simulink library "gensetMV"  (R2013a)
settings: Solver=ode3  StartTime=0.0  StopTime=10.0  RelTol=1e-3
values from neighbouring files (symbols this model uses):
  AFlowcontrol = AFhighc    (= 23)    [init_ele.m]
  AFn = 27*ones(engines,1)    [initHybrid.m]    (also in initMV.m; init_ele.m = 27)
  genset = generators(1)    [runTempCyl4S.m]
  i = i + 1    (= 2)    [DataProcessGUI1.m]    (also in NOxProcessGUI.m)
  ma0 = .2*ones(engines,1)    [initHybrid.m]    (also in initMV.m; init_ele.m = 0.2)
  nr = 1    [init_ele.m]
undefined symbols (not defined in the file or in its folder): generators, Kappa1, magnitude, pin0, swbId
libraries: goto x6, genset x2, EngineSysteSubmodel x2, simulink x1, switchboard x1
settings Model: Creator=torstebo  LastModifiedBy=yum

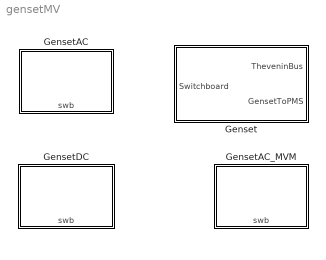
== system gensetMV ==
  Genset : Subsystem
  GensetAC : Subsystem  Tag=GensetAC  mask{genset=generators(6), swbId=3}
      mask prompts: genset "Generator set data"; swbId "SwitchboardId"
      mask Display: image(imread('figs/generator.jpg'),'center')
  GensetAC_MVM : Subsystem  Tag=GensetAC  mask{genset=generators(1), swbId=3}
      mask prompts: genset "Generator set data"; swbId "SwitchboardId"
      mask Display: image(imread('figs/generator.jpg'),'center')
  GensetDC : Subsystem  Tag=GensetDC  mask{genset=generators(1), swbId=1}
      mask prompts: genset "Generator set data"; swbId "SwitchboardId"
      mask Display: image(imread('figs/generator.jpg'),'center')

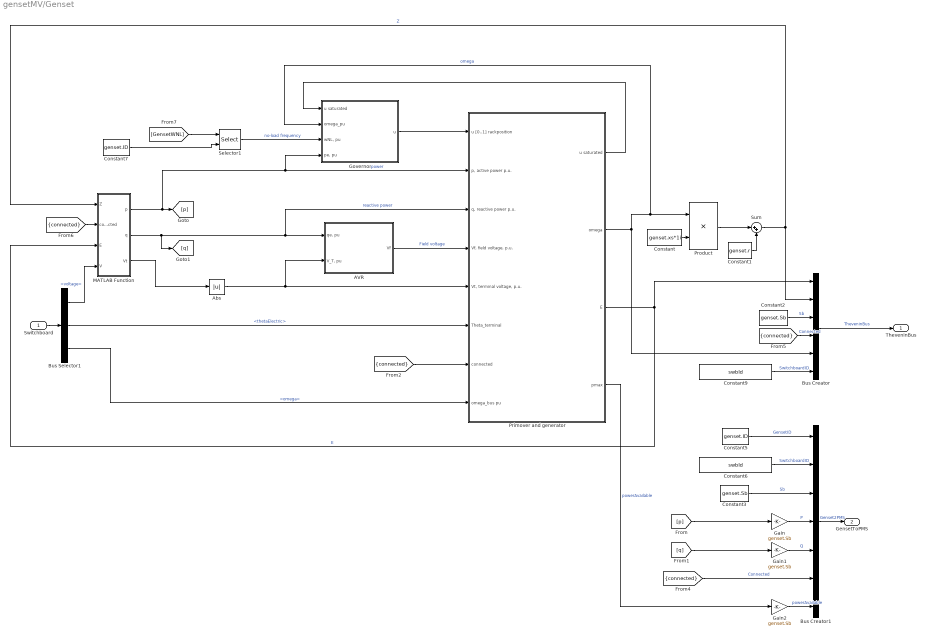
== system gensetMV/Genset ==
  Switchboard : Inport
  AVR : Subsystem
  Abs : Abs
  Bus Creator : BusCreator  Inputs='E','Z','Sb','Connected','omega','SwitchboardID'  OutDataTypeStr=Bus: TheveninBus  NonVirtualBus=on
  Bus Creator1 : BusCreator  Inputs='GensetID','SwitchboardID','Sb','P','Q','Connected','powerAvailable'  OutDataTypeStr=Bus: Genset2PMS  NonVirtualBus=on
  Bus Selector1 : BusSelector  OutputSignals=voltage,thetaElectric,omega
  Constant : Constant  Value=genset.xs*1i
  Constant1 : Constant  Value=genset.r
  Constant2 : Constant  Value=genset.Sb
  Constant3 : Constant  Value=genset.Sb
  Constant5 : Constant  Value=genset.ID  OutDataTypeStr=Inherit: Inherit via back propagation
  Constant6 : Constant  Value=swbId  OutDataTypeStr=Inherit: Inherit via back propagation
  Constant7 : Constant  Value=genset.ID  OutDataTypeStr=Inherit: Inherit via back propagation
  Constant9 : Constant  Value=swbId  OutDataTypeStr=Inherit: Inherit via back propagation
  Gain : Gain  Gain=genset.Sb
  Gain1 : Gain  Gain=genset.Sb
  Gain2 : Gain  Gain=genset.Sb
  Governor : Subsystem
  MATLAB Function : MATLAB Function  TreatAsAtomicUnit=on
  Primover and generator : Subsystem
  Product : Product
  Selector1 : Selector  IndexOptions=Index vector (port)  Indices=[nr]  OutputSizes=1
  Sum : Sum  Inputs=|++
  TheveninBus : Outport
  GensetToPMS : Outport  Port=2
  wires:
  Bus Selector1/2 -> Primover and generator/6(Theta_terminal)  "<thetaElectric>"
  Constant9/1 -> Bus Creator/6  "SwitchboardID"
  Switchboard/1 -> Bus Selector1/1
  Bus Selector1/3 -> Primover and generator/8(omega_bus pu)  "<omega>"
  MATLAB Function/3(Vt) -> Abs/1
  [connected] -> Bus Creator/4  "Connected"
  [connected] -> Bus Creator1/6  "Connected"
  [connected] -> MATLAB Function/2(connected)
  [connected] -> Primover and generator/7(connected)
  Gain2/1 -> Bus Creator1/7  "powerAvailable"
  Bus Selector1/1 -> MATLAB Function/4(V)  "<voltage>"
  Gain1/1 -> Bus Creator1/5  "Q"
  Gain/1 -> Bus Creator1/4  "P"
  Constant6/1 -> Bus Creator1/2  "SwitchboardID"
  Constant5/1 -> Bus Creator1/1  "GensetID"
  Constant3/1 -> Bus Creator1/3  "Sb"
  Selector1/1 -> Governor/3("wNL, pu")  "no-load frequency"
  AVR/1(Vf) -> Primover and generator/4("Vf, field voltage, p.u.")  "Field voltage"
  Primover and generator/1(u saturated) -> Governor/1(u saturated)
  Primover and generator/2(omega) -> Bus Creator/5, Governor/2(omega_pu), Product/1  "omega"
  Primover and generator/3(E) -> MATLAB Function/3(E), Bus Creator/1  "E"
  Governor/1(u) -> Primover and generator/1(u [0..1] rackposition)
  [GensetWNL] -> Selector1/1
  MATLAB Function/1(p) -> Primover and generator/2("p, active power p.u."), Governor/4("pe, pu"), [p]  "power"
  MATLAB Function/2(q) -> Primover and generator/3("q, reactive power p.u."), AVR/1("qe, pu"), [q]  "reactive power"
  Primover and generator/4(pmax) -> Gain2/1  "powerAvailable"
  Abs/1 -> Primover and generator/5("Vt, terminal voltage, p.u."), AVR/2("V_T, pu")
  Constant/1 -> Product/2
  Product/1 -> Sum/1
  Constant1/1 -> Sum/2
  Sum/1 -> MATLAB Function/1(Z), Bus Creator/2  "Z"
  Bus Creator/1 -> TheveninBus/1  "TheveninBus"
  Constant2/1 -> Bus Creator/3  "Sb"
  [q] -> Gain1/1
  [p] -> Gain/1
  Constant7/1 -> Selector1/2
  Bus Creator1/1 -> GensetToPMS/1  "Genset2PMS"

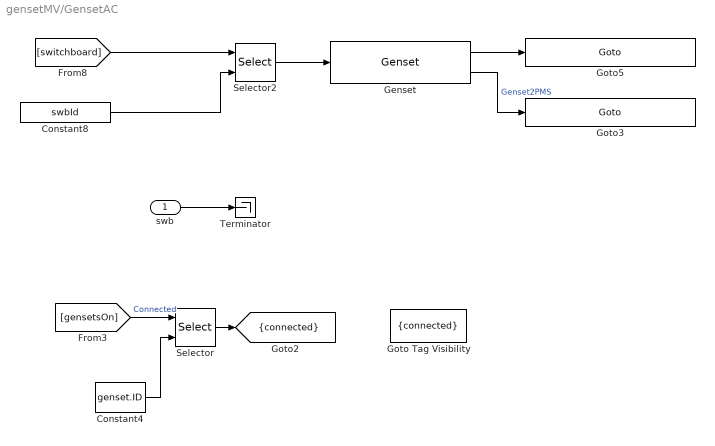
== system gensetMV/GensetAC ==
  swb : Inport
  Constant4 : Constant  Value=genset.ID  OutDataTypeStr=Inherit: Inherit via back propagation
  Constant8 : Constant  Value=swbId  OutDataTypeStr=Inherit: Inherit via back propagation
  Genset : genset/Genset
  Goto Tag Visibility : GotoTagVisibility  GotoTag=connected
  Goto3 : goto/Goto  GotoTag=sprintf('Generatorset%d',genset.ID)
  Goto5 : goto/Goto  GotoTag=sprintf('GeneratorsetElectric%d',genset.ID)
  Selector : Selector  IndexOptions=Index vector (port)  Indices=[nr]  OutputSizes=1
  Selector2 : Selector  IndexOptions=Index vector (port)  Indices=[nr]  OutputSizes=1
  Terminator : Terminator
  tag scope: connected=scoped
  wires:
  Constant8/1 -> Selector2/2
  swb/1 -> Terminator/1
  Selector/1 -> [connected]
  [gensetsOn] -> Selector/1  "Connected"
  [switchboard] -> Selector2/1
  Constant4/1 -> Selector/2
  Selector2/1 -> Genset/1
  Genset/1 -> Goto5/1
  Genset/2 -> Goto3/1  "Genset2PMS"

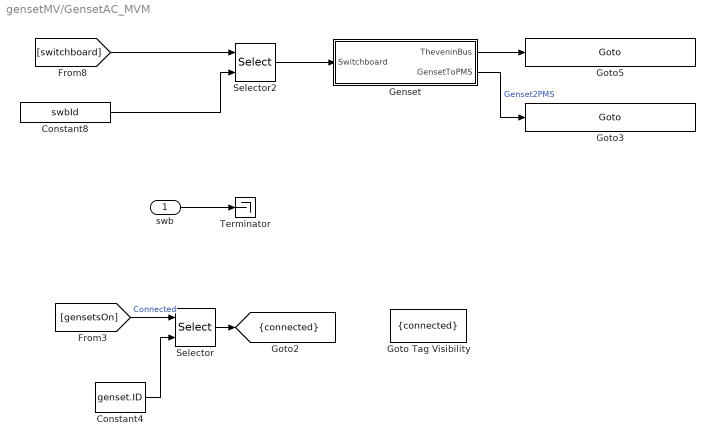
== system gensetMV/GensetAC_MVM ==
  swb : Inport
  Constant4 : Constant  Value=genset.ID  OutDataTypeStr=Inherit: Inherit via back propagation
  Constant8 : Constant  Value=swbId  OutDataTypeStr=Inherit: Inherit via back propagation
  Genset : Subsystem
  Goto Tag Visibility : GotoTagVisibility  GotoTag=connected
  Goto3 : goto/Goto  GotoTag=sprintf('Generatorset%d',genset.ID)
  Goto5 : goto/Goto  GotoTag=sprintf('GeneratorsetElectric%d',genset.ID)
  Selector : Selector  IndexOptions=Index vector (port)  Indices=[nr]  OutputSizes=1
  Selector2 : Selector  IndexOptions=Index vector (port)  Indices=[nr]  OutputSizes=1
  Terminator : Terminator
  tag scope: connected=scoped
  wires:
  Constant8/1 -> Selector2/2
  swb/1 -> Terminator/1
  Selector/1 -> [connected]
  [gensetsOn] -> Selector/1  "Connected"
  [switchboard] -> Selector2/1
  Constant4/1 -> Selector/2
  Selector2/1 -> Genset/1(Switchboard)
  Genset/1(TheveninBus) -> Goto5/1
  Genset/2(GensetToPMS) -> Goto3/1  "Genset2PMS"

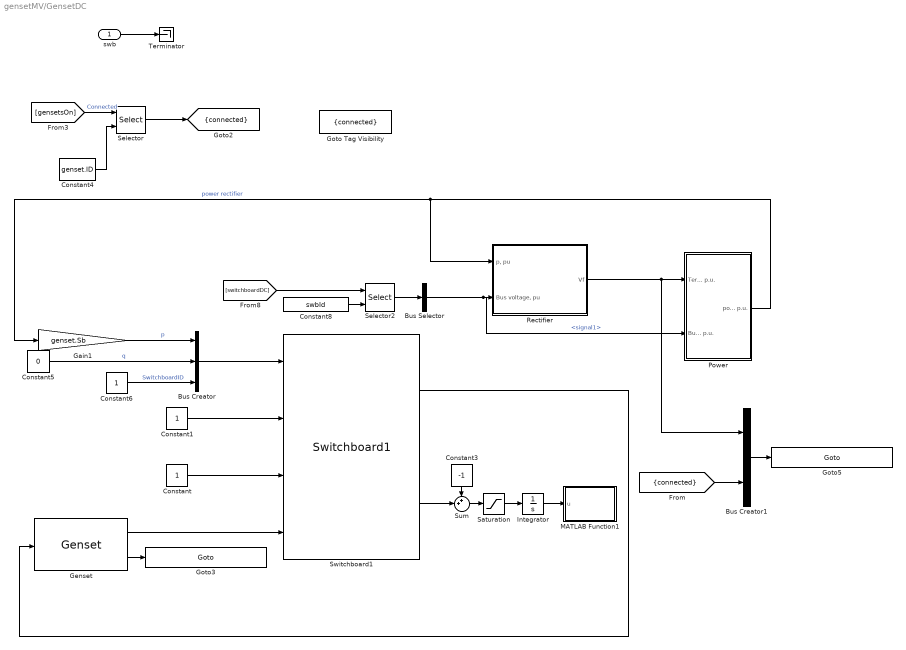
== system gensetMV/GensetDC ==
  swb : Inport
  Bus Creator : BusCreator  Inputs=3  OutDataTypeStr=Bus: powerLoadsBus
  Bus Creator1 : BusCreator  Inputs=2
  Bus Selector : BusSelector  OutputSignals=signal1
  Constant : Constant
  Constant1 : Constant
  Constant3 : Constant  Value=-1
  Constant4 : Constant  Value=genset.ID  OutDataTypeStr=Inherit: Inherit via back propagation
  Constant5 : Constant  Value=0
  Constant6 : Constant
  Constant8 : Constant  Value=swbId  OutDataTypeStr=Inherit: Inherit via back propagation
  Gain1 : Gain  Gain=genset.Sb
  Genset : genset/Genset
  Goto Tag Visibility : GotoTagVisibility  GotoTag=connected
  Goto3 : goto/Goto  GotoTag=sprintf('GeneratorsetDC%d',genset.ID)
  Goto5 : goto/Goto  GotoTag=sprintf('GeneratorsetElectricDC%d',genset.ID)
  Integrator : Integrator
  MATLAB Function1 : MATLAB Function  TreatAsAtomicUnit=on
  Power : Subsystem
  Rectifier : Subsystem
  Saturation : Saturate  UpperLimit=0  LowerLimit=-1
  Selector : Selector  IndexOptions=Index vector (port)  Indices=[nr]  OutputSizes=1
  Selector2 : Selector  IndexOptions=Index vector (port)  Indices=[nr]  OutputSizes=1
  Sum : Sum  Inputs=++|
  Switchboard1 : switchboard/Switchboard1
  Terminator : Terminator
  tag scope: connected=scoped
  wires:
  Constant8/1 -> Selector2/2
  swb/1 -> Terminator/1
  Selector/1 -> [connected]
  [gensetsOn] -> Selector/1  "Connected"
  [switchboardDC] -> Selector2/1
  Constant4/1 -> Selector/2
  Selector2/1 -> Bus Selector/1
  Rectifier/1(Vf) -> Bus Creator1/1, Power/1(Terminal Voltage p.u.)
  Power/1(power p.u.) -> Rectifier/1("p, pu"), Gain1/1  "power rectifier"
  Bus Selector/1 -> Power/2(Bus Voltage p.u.), Rectifier/2("Bus voltage, pu")  "<signal1>"
  Gain1/1 -> Bus Creator/1  "p"
  Bus Creator/1 -> Switchboard1/1
  Constant3/1 -> Sum/1
  Constant5/1 -> Bus Creator/2  "q"
  Integrator/1 -> MATLAB Function1/1(u)
  Genset/1 -> Switchboard1/4
  Constant/1 -> Switchboard1/3
  Sum/1 -> Saturation/1
  Saturation/1 -> Integrator/1
  Switchboard1/1 -> Genset/1
  Constant6/1 -> Bus Creator/3  "SwitchboardID"
  Switchboard1/2 -> Sum/2
  Constant1/1 -> Switchboard1/2
  Bus Creator1/1 -> Goto5/1
  [connected] -> Bus Creator1/2
  Genset/2 -> Goto3/1

== system gensetMV/Genset/AVR ==
  "qe, pu" : Inport
  "V_T, pu" : Inport  Port=2
  Constant : Constant
  Constant7 : Constant  Value=genset.ID  OutDataTypeStr=Inherit: Inherit via back propagation
  Gain : Gain  Gain=genset.avr.droop
  Low pass filter : Subsystem
  PI controller : Subsystem
  Product : Product  RndMeth=Zero
  Selector1 : Selector  IndexOptions=Index vector (port)  Indices=[nr]  OutputSizes=1
  Sum1 : Sum  Inputs=|+-
  Sum3 : Sum  Inputs=|+-
  Vf : Outport
  wires:
  Selector1/1 -> Product/1  "no-load frequency"
  [GensetVNL] -> Selector1/1
  Constant7/1 -> Selector1/2
  PI controller/1(vf) -> Low pass filter/1(V)
  Sum1/1 -> PI controller/1(e)
  "qe, pu"/1 -> Gain/1
  "V_T, pu"/1 -> Sum1/2
  Constant/1 -> Sum3/1
  Gain/1 -> Sum3/2
  Sum3/1 -> Product/2
  Product/1 -> Sum1/1
  Low pass filter/1(Vold) -> Vf/1

== system gensetMV/Genset/Governor ==
  u saturated : Inport
  omega_pu : Inport  Port=2
  "wNL, pu" : Inport  Port=3
  "pe, pu" : Inport  Port=4
  Constant : Constant
  Gain : Gain  Gain=genset.governor.droop
  PID controller : Subsystem
  Product : Product  RndMeth=Zero
  Sum : Sum  Inputs=|+-
  Sum1 : Sum  Inputs=|+-
  u : Outport
  wires:
  PID controller/1(u) -> u/1  "u"
  Gain/1 -> Sum1/2
  Sum/1 -> PID controller/1(e)
  Product/1 -> Sum/1
  "wNL, pu"/1 -> Product/1
  Constant/1 -> Sum1/1
  Sum1/1 -> Product/2
  u saturated/1 -> PID controller/3(u saturated)
  "pe, pu"/1 -> Gain/1
  omega_pu/1 -> Sum/2, PID controller/2(omega_pu)

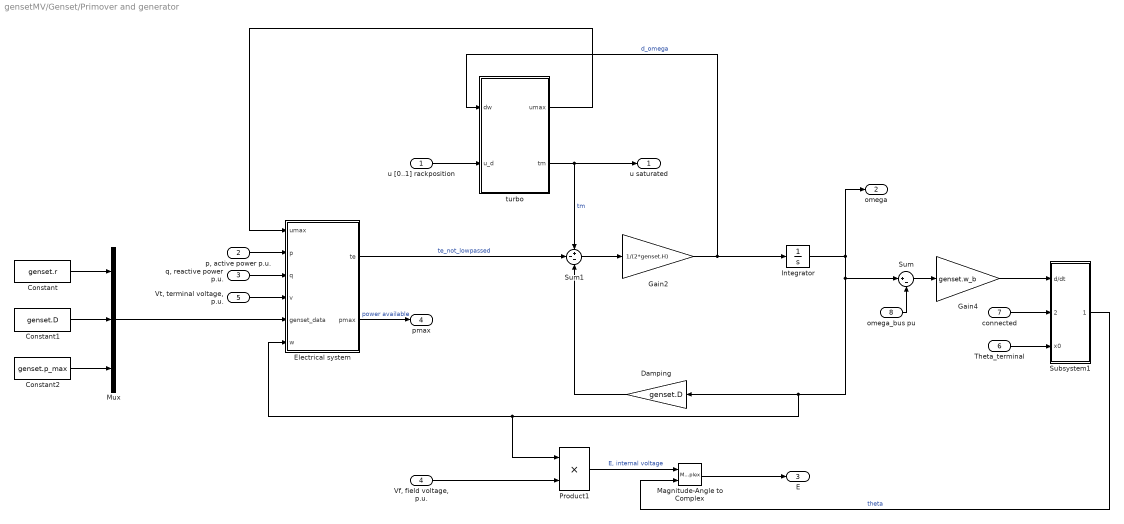
== system gensetMV/Genset/Primover and generator ==
  u [0..1] rackposition : Inport
  "p, active power p.u." : Inport  Port=2
  "q, reactive power p.u." : Inport  Port=3
  "Vf, field voltage, p.u." : Inport  Port=4
  "Vt, terminal voltage, p.u." : Inport  Port=5
  Theta_terminal : Inport  Port=6
  connected : Inport  Port=7
  omega_bus pu : Inport  Port=8
  Constant : Constant  Value=genset.r
  Constant1 : Constant  Value=genset.D
  Constant2 : Constant  Value=genset.p_max
  Damping : Gain  Gain=genset.D
  Electrical system : MATLAB Function  TreatAsAtomicUnit=on
  Gain2 : Gain  Gain=1/(2*genset.H)
  Gain4 : Gain  Gain=genset.w_b
  Integrator : Integrator  InitialCondition=genset.omega0
  Magnitude-Angle to Complex : MagnitudeAngleToComplex
  Mux : Mux  Inputs=3
  Product1 : Product  Inputs=**  RndMeth=Zero
  Subsystem1 : Subsystem
  Sum : Sum  Inputs=|+-
  Sum1 : Sum  Inputs=+--
  turbo : Subsystem
  u saturated : Outport
  omega : Outport  Port=2
  E : Outport  Port=3
  pmax : Outport  Port=4
  wires:
  omega_bus pu/1 -> Sum/2
  Sum/1 -> Gain4/1
  u [0..1] rackposition/1 -> turbo/2(u_d)
  turbo/2(tm) -> u saturated/1, Sum1/1  "tm"
  Product1/1 -> Magnitude-Angle to Complex/1  "E, internal voltage"
  Subsystem1/1(Out1) -> Magnitude-Angle to Complex/2  "theta"
  Gain4/1 -> Subsystem1/1(d/dt)
  Sum1/1 -> Gain2/1
  Gain2/1 -> turbo/1(dw), Integrator/1  "d_omega"
  "Vf, field voltage, p.u."/1 -> Product1/2
  "p, active power p.u."/1 -> Electrical system/2(p)
  Electrical system/1(te) -> Sum1/2  "te_not_lowpassed"
  "Vt, terminal voltage, p.u."/1 -> Electrical system/4(v)
  "q, reactive power p.u."/1 -> Electrical system/3(q)
  Damping/1 -> Sum1/3
  connected/1 -> Subsystem1/2(reset)
  Integrator/1 -> Sum/1, Damping/1, Product1/1, Electrical system/6(w), omega/1
  Theta_terminal/1 -> Subsystem1/3(x0)
  turbo/1(umax) -> Electrical system/1(umax)
  Electrical system/2(pmax) -> pmax/1  "power available"
  Magnitude-Angle to Complex/1 -> E/1
  Constant/1 -> Mux/1
  Constant1/1 -> Mux/2
  Constant2/1 -> Mux/3
  Mux/1 -> Electrical system/5(genset_data)

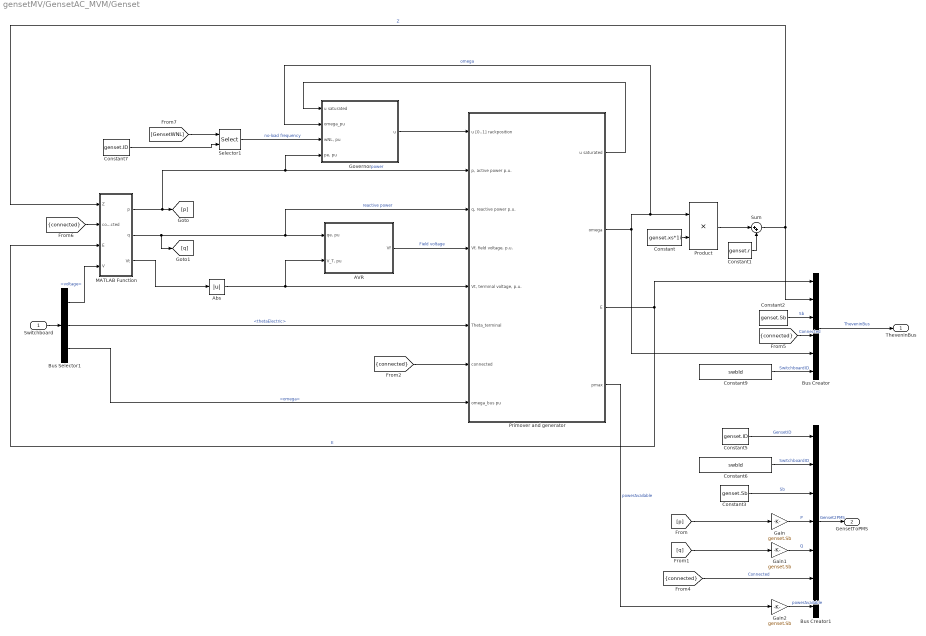
== system gensetMV/GensetAC_MVM/Genset ==
  Switchboard : Inport
  AVR : Subsystem
  Abs : Abs
  Bus Creator : BusCreator  Inputs='E','Z','Sb','Connected','omega','SwitchboardID'  OutDataTypeStr=Bus: TheveninBus  NonVirtualBus=on
  Bus Creator1 : BusCreator  Inputs='GensetID','SwitchboardID','Sb','P','Q','Connected','powerAvailable'  OutDataTypeStr=Bus: Genset2PMS  NonVirtualBus=on
  Bus Selector1 : BusSelector  OutputSignals=voltage,thetaElectric,omega
  Constant : Constant  Value=genset.xs*1i
  Constant1 : Constant  Value=genset.r
  Constant2 : Constant  Value=genset.Sb
  Constant3 : Constant  Value=genset.Sb
  Constant5 : Constant  Value=genset.ID  OutDataTypeStr=Inherit: Inherit via back propagation
  Constant6 : Constant  Value=swbId  OutDataTypeStr=Inherit: Inherit via back propagation
  Constant7 : Constant  Value=genset.ID  OutDataTypeStr=Inherit: Inherit via back propagation
  Constant9 : Constant  Value=swbId  OutDataTypeStr=Inherit: Inherit via back propagation
  Gain : Gain  Gain=genset.Sb
  Gain1 : Gain  Gain=genset.Sb
  Gain2 : Gain  Gain=genset.Sb
  Governor : Subsystem
  MATLAB Function : MATLAB Function  TreatAsAtomicUnit=on
  Primover and generator : Subsystem
  Product : Product
  Selector1 : Selector  IndexOptions=Index vector (port)  Indices=[nr]  OutputSizes=1
  Sum : Sum  Inputs=|++
  TheveninBus : Outport
  GensetToPMS : Outport  Port=2
  wires:
  Bus Creator1/1 -> GensetToPMS/1  "Genset2PMS"
  Constant7/1 -> Selector1/2
  [p] -> Gain/1
  [q] -> Gain1/1
  Constant2/1 -> Bus Creator/3  "Sb"
  Bus Creator/1 -> TheveninBus/1  "TheveninBus"
  Sum/1 -> Bus Creator/2, MATLAB Function/1(Z)  "Z"
  Constant1/1 -> Sum/2
  Product/1 -> Sum/1
  Constant/1 -> Product/2
  Abs/1 -> AVR/2("V_T, pu"), Primover and generator/5("Vt, terminal voltage, p.u.")
  Primover and generator/4(pmax) -> Gain2/1  "powerAvailable"
  MATLAB Function/2(q) -> [q], AVR/1("qe, pu"), Primover and generator/3("q, reactive power p.u.")  "reactive power"
  MATLAB Function/1(p) -> [p], Governor/4("pe, pu"), Primover and generator/2("p, active power p.u.")  "power"
  [GensetWNL] -> Selector1/1
  Governor/1(u) -> Primover and generator/1(u [0..1] rackposition)
  Primover and generator/3(E) -> Bus Creator/1, MATLAB Function/3(E)  "E"
  Primover and generator/2(omega) -> Product/1, Governor/2(omega_pu), Bus Creator/5  "omega"
  Primover and generator/1(u saturated) -> Governor/1(u saturated)
  AVR/1(Vf) -> Primover and generator/4("Vf, field voltage, p.u.")  "Field voltage"
  Selector1/1 -> Governor/3("wNL, pu")  "no-load frequency"
  Constant3/1 -> Bus Creator1/3  "Sb"
  Constant5/1 -> Bus Creator1/1  "GensetID"
  Constant6/1 -> Bus Creator1/2  "SwitchboardID"
  Gain/1 -> Bus Creator1/4  "P"
  Gain1/1 -> Bus Creator1/5  "Q"
  Bus Selector1/1 -> MATLAB Function/4(V)  "<voltage>"
  Gain2/1 -> Bus Creator1/7  "powerAvailable"
  [connected] -> Primover and generator/7(connected)
  [connected] -> MATLAB Function/2(connected)
  [connected] -> Bus Creator1/6  "Connected"
  [connected] -> Bus Creator/4  "Connected"
  MATLAB Function/3(Vt) -> Abs/1
  Bus Selector1/3 -> Primover and generator/8(omega_bus pu)  "<omega>"
  Switchboard/1 -> Bus Selector1/1
  Constant9/1 -> Bus Creator/6  "SwitchboardID"
  Bus Selector1/2 -> Primover and generator/6(Theta_terminal)  "<thetaElectric>"

== system gensetMV/GensetDC/Power ==
  Terminal Voltage p.u. : Inport
  Bus Voltage p.u. : Inport  Port=2
  Gain : Gain  Gain=1/genset.rectifier.r
  Product : Product
  Sum1 : Sum  Inputs=+|-
  power p.u. : Outport
  wires:
  Gain/1 -> Product/2  "current"
  Sum1/1 -> Gain/1
  Bus Voltage p.u./1 -> Sum1/2
  Terminal Voltage p.u./1 -> Product/1, Sum1/1
  Product/1 -> power p.u./1

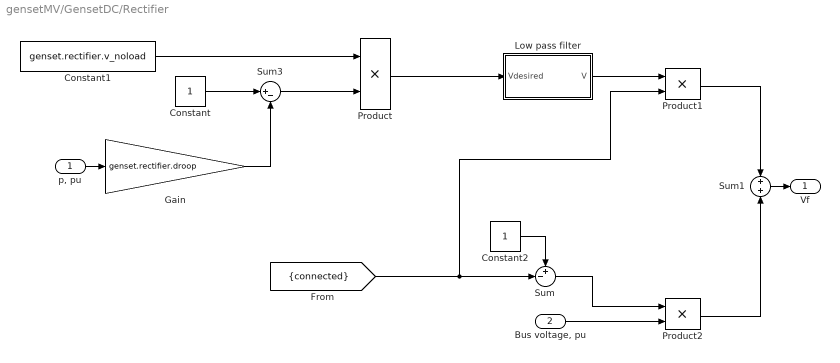
== system gensetMV/GensetDC/Rectifier ==
  "p, pu" : Inport
  "Bus voltage, pu" : Inport  Port=2
  Constant : Constant
  Constant1 : Constant  Value=genset.rectifier.v_noload
  Constant2 : Constant
  Gain : Gain  Gain=genset.rectifier.droop
  Low pass filter : Subsystem
  Product : Product  RndMeth=Zero
  Product1 : Product
  Product2 : Product
  Sum : Sum  Inputs=+-|
  Sum1 : Sum
  Sum3 : Sum  Inputs=|+-
  Vf : Outport
  wires:
  Product/1 -> Low pass filter/1(Vdesired)
  "p, pu"/1 -> Gain/1
  Constant1/1 -> Product/1
  Constant/1 -> Sum3/1
  Gain/1 -> Sum3/2
  Sum3/1 -> Product/2
  Low pass filter/1(V) -> Product1/1
  "Bus voltage, pu"/1 -> Product2/2
  [connected] -> Product1/2, Sum/2
  Constant2/1 -> Sum/1
  Sum/1 -> Product2/1
  Product2/1 -> Sum1/2
  Product1/1 -> Sum1/1
  Sum1/1 -> Vf/1

== system gensetMV/Genset/AVR/Low pass filter ==
  V : Inport
  Gain : Gain  Gain=1/genset.avr.T
  Integrator : Integrator  InitialCondition=genset.avr.v0
  Sum : Sum  Inputs=|+-
  Vold : Outport
  wires:
  Integrator/1 -> Vold/1, Sum/2
  V/1 -> Sum/1
  Sum/1 -> Gain/1
  Gain/1 -> Integrator/1

== system gensetMV/Genset/AVR/PI controller ==
  e : Inport
  Gain : Gain  Gain=genset.avr.Ki
  Gain1 : Gain  Gain=genset.avr.Kp
  Integrator : Integrator  DisableCoverage=on  InitialCondition=genset.avr.v0
  Saturation : Saturate  UpperLimit=genset.avr.max_fv  LowerLimit=genset.avr.min_fv  LinearizeAsGain=off  OutMin=genset.avr.min_fv  OutMax=genset.avr.max_fv  OutDataTypeStr=Inherit: Inherit via back propagation
  Sum : Sum  Inputs=+|+
  vf : Outport
  wires:
  Saturation/1 -> vf/1
  Sum/1 -> Saturation/1
  e/1 -> Gain/1, Gain1/1
  Integrator/1 -> Sum/2
  Gain1/1 -> Sum/1
  Gain/1 -> Integrator/1

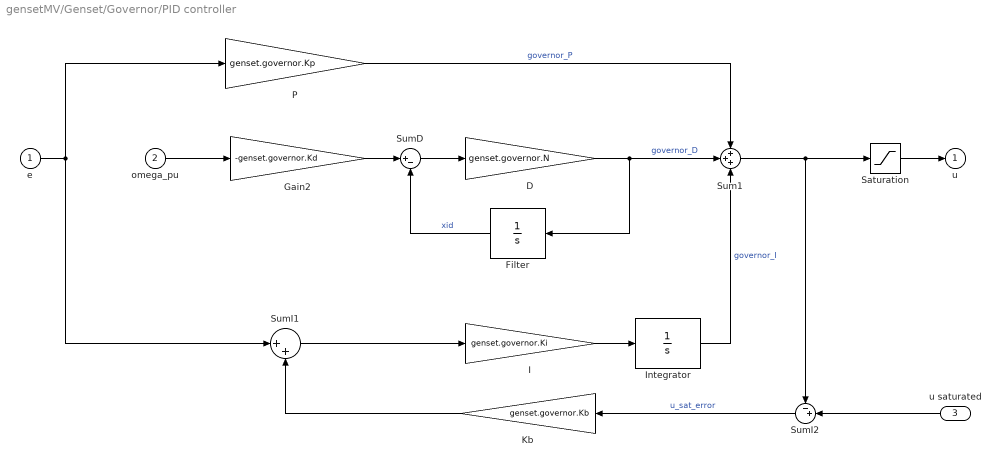
== system gensetMV/Genset/Governor/PID controller ==
  e : Inport  PortDimensions=1
  omega_pu : Inport  Port=2  PortDimensions=1
  u saturated : Inport  Port=3  PortDimensions=1
  D : Gain  DisableCoverage=on  Gain=genset.governor.N
  Filter : Integrator  DisableCoverage=on  InitialCondition=-genset.omega0*genset.governor.Kd
  Gain2 : Gain  Gain=-genset.governor.Kd
  I : Gain  Gain=genset.governor.Ki
  Integrator : Integrator  DisableCoverage=on  InitialCondition=genset.u0
  Kb : Gain  DisableCoverage=on  Gain=genset.governor.Kb  ParamDataTypeStr=Inherit: Inherit from 'Gain'
  P : Gain  Gain=genset.governor.Kp
  Saturation : Saturate  UpperLimit=genset.u_max  LowerLimit=genset.u_min  LinearizeAsGain=off  OutMin=genset.u_min  OutMax=genset.u_max  OutDataTypeStr=Inherit: Inherit via back propagation
  Sum1 : Sum  Inputs=+++
  SumD : Sum  DisableCoverage=on  Inputs=|+-
  SumI1 : Sum  DisableCoverage=on  Inputs=|++
  SumI2 : Sum  DisableCoverage=on  Inputs=-+|
  u : Outport  PortDimensions=1  InitialOutput=0
  wires:
  Integrator/1 -> Sum1/3  "governor_I"
  D/1 -> Sum1/2, Filter/1  "governor_D"
  omega_pu/1 -> Gain2/1
  e/1 -> P/1, SumI1/1
  P/1 -> Sum1/1  "governor_P"
  Saturation/1 -> u/1
  Filter/1 -> SumD/2  "xid"
  SumD/1 -> D/1
  Gain2/1 -> SumD/1
  Sum1/1 -> Saturation/1, SumI2/1
  SumI2/1 -> Kb/1  "u_sat_error"
  Kb/1 -> SumI1/2
  u saturated/1 -> SumI2/2
  SumI1/1 -> I/1
  I/1 -> Integrator/1

== system gensetMV/Genset/Primover and generator/Subsystem1 ==
  d/dt : Inport
  reset : Inport  Port=2
  x0 : Inport  Port=3
  Gain : Gain  Gain=1000
  Integrator : Integrator  InitialCondition=genset.theta0
  MATLAB Function : MATLAB Function  TreatAsAtomicUnit=on
  Sum : Sum  Inputs=-|+
  Switch : Switch  Threshold=1
  Out1 : Outport
  wires:
  Integrator/1 -> Out1/1, Sum/1
  reset/1 -> Switch/2
  x0/1 -> Sum/2
  Sum/1 -> MATLAB Function/1(u)
  Gain/1 -> Switch/3
  MATLAB Function/1(y) -> Gain/1
  d/dt/1 -> Switch/1
  Switch/1 -> Integrator/1

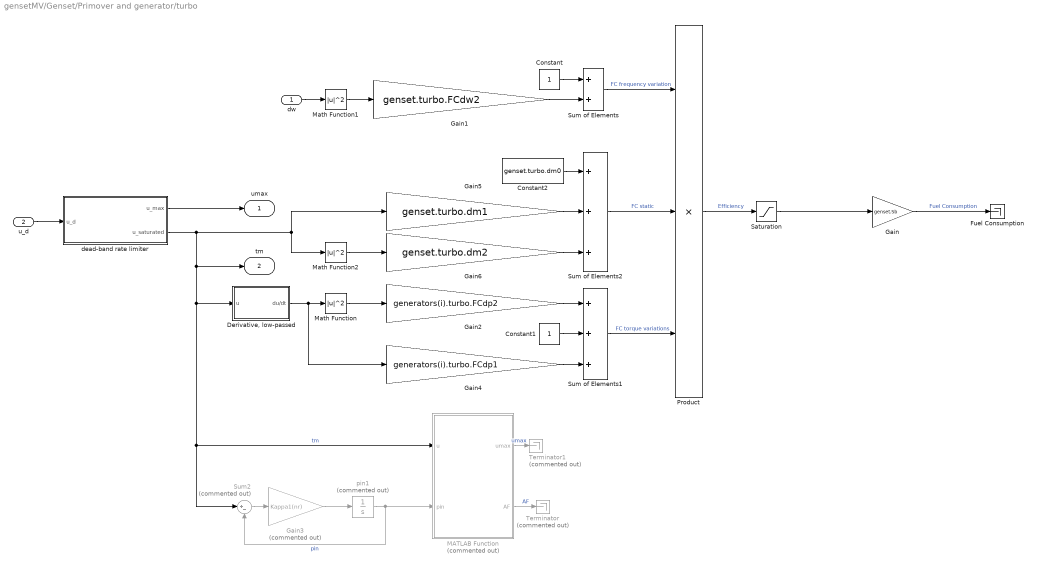
== system gensetMV/Genset/Primover and generator/turbo ==
  dw : Inport
  u_d : Inport  Port=2
  Constant : Constant
  Constant1 : Constant
  Constant2 : Constant  Value=genset.turbo.dm0
  "Derivative, low-passed" : Subsystem
      settings: MinAlgLoopOccurrences=on
  Fuel Consumption : Terminator
  Gain : Gain  Gain=genset.Sb
  Gain1 : Gain  Gain=genset.turbo.FCdw2
  Gain2 : Gain  Gain=generators(i).turbo.FCdp2
  Gain3 : Gain  Commented=on  Gain=Kappa1(nr)
  Gain4 : Gain  Gain=generators(i).turbo.FCdp1
  Gain5 : Gain  Gain=genset.turbo.dm1
  Gain6 : Gain  Gain=genset.turbo.dm2
  MATLAB Function : MATLAB Function  Commented=on  TreatAsAtomicUnit=on
  Math Function : Math  Operator=magnitude^2  SaturateOnIntegerOverflow=on
  Math Function1 : Math  Operator=magnitude^2  SaturateOnIntegerOverflow=on
  Math Function2 : Math  Operator=magnitude^2  SaturateOnIntegerOverflow=on
  Product : Product  Inputs=3  RndMeth=Zero
  Saturation : Saturate  UpperLimit=genset.turbo.FCmax  LowerLimit=0
  Sum of Elements : Sum
  Sum of Elements1 : Sum  Inputs=+++
  Sum of Elements2 : Sum  Inputs=+++
  Sum2 : Sum  Commented=on  Inputs=|+-
  Terminator : Terminator  Commented=on
  Terminator1 : Terminator  Commented=on
  dead-band rate limiter : Subsystem  mask(Rate limiter for diesel engines){umax=genset.u_max, umin=genset.u_min}
      mask prompts: umax "Static maximum torque"; umin "Static minimum torque"
      mask help:
      | Allows the input to change within a delta limit, however if the input
      | changes more than this range will the input be saturated by a rate limiter.
  pin1 : Integrator  Commented=on  InitialCondition=pin0(nr)
  umax : Outport
  tm : Outport  Port=2
  wires:
  Gain/1 -> Fuel Consumption/1  "Fuel Consumption"
  Saturation/1 -> Gain/1
  Product/1 -> Saturation/1  "Efficiency"
  Sum of Elements/1 -> Product/1  "FC frequency variation"
  Sum of Elements2/1 -> Product/2  "FC static"
  Sum of Elements1/1 -> Product/3  "FC torque variations"
  Math Function2/1 -> Gain6/1
  Constant2/1 -> Sum of Elements2/1
  Gain5/1 -> Sum of Elements2/2
  Gain6/1 -> Sum of Elements2/3
  Constant1/1 -> Sum of Elements1/2
  Gain4/1 -> Sum of Elements1/3
  Gain2/1 -> Sum of Elements1/1
  Constant/1 -> Sum of Elements/1
  Gain1/1 -> Sum of Elements/2
  Math Function/1 -> Gain2/1
  Math Function1/1 -> Gain1/1
  "Derivative, low-passed"/1(du/dt) -> Math Function/1, Gain4/1
  pin1/1 -> MATLAB Function/2(pin), Sum2/2  "pin"
  Sum2/1 -> Gain3/1
  Gain3/1 -> pin1/1
  dead-band rate limiter/2(u_saturated) -> tm/1, Sum2/1, MATLAB Function/1(u), "Derivative, low-passed"/1(u), Gain5/1, Math Function2/1  "tm"
  u_d/1 -> dead-band rate limiter/1(u_d)
  MATLAB Function/2(AF) -> Terminator/1  "AF"
  dw/1 -> Math Function1/1
  MATLAB Function/1(umax) -> Terminator1/1  "umax"
  dead-band rate limiter/1(u_max) -> umax/1

== system gensetMV/GensetAC_MVM/Genset/AVR ==
  "qe, pu" : Inport
  "V_T, pu" : Inport  Port=2
  Constant : Constant
  Constant7 : Constant  Value=genset.ID  OutDataTypeStr=Inherit: Inherit via back propagation
  Gain : Gain  Gain=genset.avr.droop
  Low pass filter : Subsystem
  PI controller : Subsystem
  Product : Product  RndMeth=Zero
  Selector1 : Selector  IndexOptions=Index vector (port)  Indices=[nr]  OutputSizes=1
  Sum1 : Sum  Inputs=|+-
  Sum3 : Sum  Inputs=|+-
  Vf : Outport
  wires:
  Low pass filter/1(Vold) -> Vf/1
  Product/1 -> Sum1/1
  Sum3/1 -> Product/2
  Gain/1 -> Sum3/2
  Constant/1 -> Sum3/1
  "V_T, pu"/1 -> Sum1/2
  "qe, pu"/1 -> Gain/1
  Sum1/1 -> PI controller/1(e)
  PI controller/1(vf) -> Low pass filter/1(V)
  Constant7/1 -> Selector1/2
  [GensetVNL] -> Selector1/1
  Selector1/1 -> Product/1  "no-load frequency"

== system gensetMV/GensetAC_MVM/Genset/Governor ==
  u saturated : Inport
  omega_pu : Inport  Port=2
  "wNL, pu" : Inport  Port=3
  "pe, pu" : Inport  Port=4
  Constant : Constant
  Gain : Gain  Gain=genset.governor.droop
  PID controller : Subsystem
  Product : Product  RndMeth=Zero
  Sum : Sum  Inputs=|+-
  Sum1 : Sum  Inputs=|+-
  u : Outport
  wires:
  omega_pu/1 -> PID controller/2(omega_pu), Sum/2
  "pe, pu"/1 -> Gain/1
  u saturated/1 -> PID controller/3(u saturated)
  Sum1/1 -> Product/2
  Constant/1 -> Sum1/1
  "wNL, pu"/1 -> Product/1
  Product/1 -> Sum/1
  Sum/1 -> PID controller/1(e)
  Gain/1 -> Sum1/2
  PID controller/1(u) -> u/1  "u"

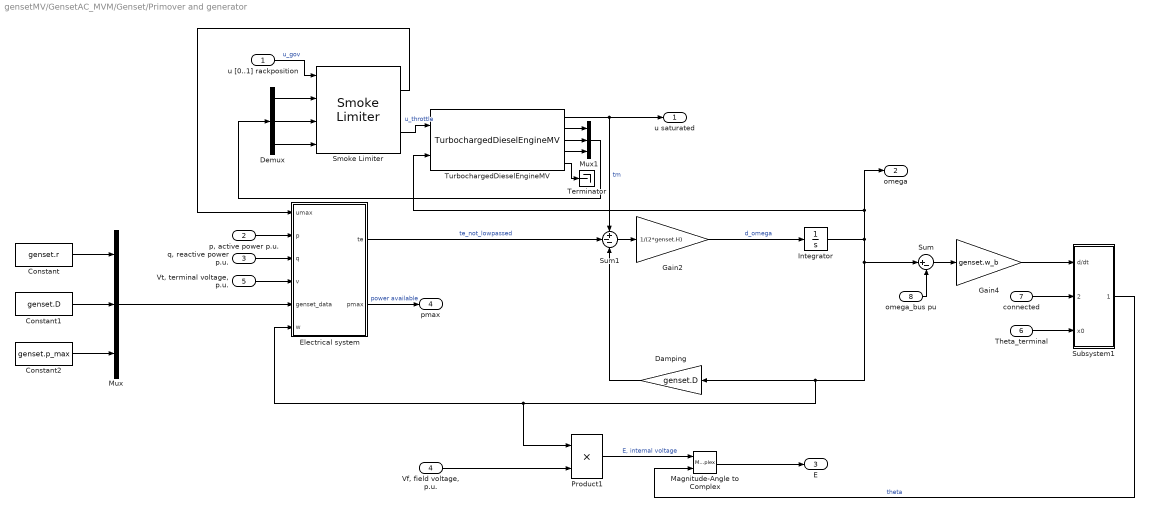
== system gensetMV/GensetAC_MVM/Genset/Primover and generator ==
  u [0..1] rackposition : Inport
  "p, active power p.u." : Inport  Port=2
  "q, reactive power p.u." : Inport  Port=3
  "Vf, field voltage, p.u." : Inport  Port=4
  "Vt, terminal voltage, p.u." : Inport  Port=5
  Theta_terminal : Inport  Port=6
  connected : Inport  Port=7
  omega_bus pu : Inport  Port=8
  Constant : Constant  Value=genset.r
  Constant1 : Constant  Value=genset.D
  Constant2 : Constant  Value=genset.p_max
  Damping : Gain  Gain=genset.D
  Demux : Demux  Outputs=3
  Electrical system : MATLAB Function  TreatAsAtomicUnit=on
  Gain2 : Gain  Gain=1/(2*genset.H)
  Gain4 : Gain  Gain=genset.w_b
  Integrator : Integrator  InitialCondition=genset.omega0
  Magnitude-Angle to Complex : MagnitudeAngleToComplex
  Mux : Mux  Inputs=3
  Mux1 : Mux  Inputs=3
  Product1 : Product  Inputs=**  RndMeth=Zero
  Smoke Limiter : EngineSysteSubmodel/Smoke Limiter  fs=genset.eng.fs  Vd=genset.eng.vD  F_max=genset.eng.fMax  m_f_cyc_max=genset.eng.mFCycMax
  Subsystem1 : Subsystem
  Sum : Sum  Inputs=|+-
  Sum1 : Sum  Inputs=+--
  Terminator : Terminator
  TurbochargedDieselEngineMV : EngineSysteSubmodel/TurbochargedDieselEngineMV  fs=genset.eng.fs  lHV=genset.eng.LHV  sFC=genset.eng.SFC  mFCycMax=genset.eng.mFCycMax  tPe=genset.eng.tPe  vD=genset.eng.vD  peNom=genset.eng.powNom  volEffCoeff1=genset.eng.volEff1  volEffCoeff2=genset.eng.volEff2  nStroke=genset.eng.nStroke  c1=genset.eng.C1  p_a_inf=genset.eng.pAInf  Pe0=genset.eng.powL0*genset.eng.powNom  omegaENom=genset.eng.omegaENom  tqShaftNom=genset.eng.tqShaftNom  jTc=genset.eng.jTC  compFlowMap=genset.eng.compFlowMap  compEffMap=genset.eng.compEffMap  prRep=genset.eng.prRep  n288Rep=genset.eng.n288Rep  npr=genset.eng.npr  nsp=genset.eng.nsp  flowCoeffTurb=genset.eng.flowCoeffTurb  dWheelTurb=genset.eng.dTurbWheel  ucOpt=genset.eng.ucOpt  effTurbMax=genset.eng.effTurbMax  tempRef=genset.eng.tempRef  omegat0=genset.eng.omegaT0  VPipeAturb=genset.eng.vPipeAComp  m0PipeAturb=genset.eng.m0PipeAComp  e0PipeAturb=genset.eng.e0PipeAComp  mb0PipeAturb=genset.eng.mb0PipeAComp  Cd=genset.eng.cdCool  AAirPath=genset.eng.aAirPath  dmCW=genset.eng.dmCW  coeffTCWK=genset.eng.coeffKTCW  cpCW=genset.eng.cpCW  dCWPipe=genset.eng.dPipeCW  tempCW=genset.eng.tCW  vAR=genset.eng.vAR  m0AR=genset.eng.m0AR  e0AR=genset.eng.E0AR  mb0AR=genset.eng.mb0AR  vER=genset.eng.vER  m0ER=genset.eng.m0ER  d0ER=genset.eng.E0ER  mb0ER=genset.eng.mb0ER  tempAmb=genset.eng.tAmb  pAmb=genset.eng.pAmb  fAmb=genset.eng.fAmb  pBack=genset.eng.pBack
  u saturated : Outport
  omega : Outport  Port=2
  E : Outport  Port=3
  pmax : Outport  Port=4
  wires:
  TurbochargedDieselEngineMV/1 -> Sum1/1, u saturated/1  "tm"
  Mux/1 -> Electrical system/5(genset_data)
  Constant2/1 -> Mux/3
  Constant1/1 -> Mux/2
  Constant/1 -> Mux/1
  Magnitude-Angle to Complex/1 -> E/1
  Electrical system/2(pmax) -> pmax/1  "power available"
  Smoke Limiter/2 -> TurbochargedDieselEngineMV/1  "u_throttle"
  Theta_terminal/1 -> Subsystem1/3(x0)
  Integrator/1 -> Sum/1, Electrical system/6(w), Product1/1, Damping/1, omega/1, TurbochargedDieselEngineMV/2
  connected/1 -> Subsystem1/2(reset)
  Damping/1 -> Sum1/3
  "q, reactive power p.u."/1 -> Electrical system/3(q)
  "Vt, terminal voltage, p.u."/1 -> Electrical system/4(v)
  Electrical system/1(te) -> Sum1/2  "te_not_lowpassed"
  "p, active power p.u."/1 -> Electrical system/2(p)
  "Vf, field voltage, p.u."/1 -> Product1/2
  Gain2/1 -> Integrator/1  "d_omega"
  Sum1/1 -> Gain2/1
  Gain4/1 -> Subsystem1/1(d/dt)
  Subsystem1/1(Out1) -> Magnitude-Angle to Complex/2  "theta"
  Product1/1 -> Magnitude-Angle to Complex/1  "E, internal voltage"
  u [0..1] rackposition/1 -> Smoke Limiter/1  "u_gov"
  Sum/1 -> Gain4/1
  omega_bus pu/1 -> Sum/2
  Smoke Limiter/1 -> Electrical system/1(umax)
  TurbochargedDieselEngineMV/2 -> Mux1/1
  TurbochargedDieselEngineMV/3 -> Mux1/2
  TurbochargedDieselEngineMV/4 -> Mux1/3
  Mux1/1 -> Demux/1
  Demux/1 -> Smoke Limiter/2
  Demux/2 -> Smoke Limiter/3
  Demux/3 -> Smoke Limiter/4
  TurbochargedDieselEngineMV/5 -> Terminator/1

== system gensetMV/GensetDC/Rectifier/Low pass filter ==
  Vdesired : Inport
  Gain : Gain  Gain=1/genset.rectifier.T
  Integrator : Integrator  InitialCondition=genset.rectifier.v0
  Sum : Sum  Inputs=|+-
  V : Outport
  wires:
  Integrator/1 -> V/1, Sum/2
  Vdesired/1 -> Sum/1
  Sum/1 -> Gain/1
  Gain/1 -> Integrator/1

== system gensetMV/Genset/Primover and generator/turbo/Derivative, low-passed ==
  u : Inport
  Gain : Gain  Gain=10
  Integrator : Integrator  InitialCondition=genset.u0
  Sum : Sum  Inputs=|+-
  du/dt : Outport
  wires:
  Sum/1 -> Gain/1
  Integrator/1 -> Sum/2
  Gain/1 -> du/dt/1, Integrator/1
  u/1 -> Sum/1

== system gensetMV/Genset/Primover and generator/turbo/dead-band rate limiter ==
  u_d : Inport
  Constant : Constant  Value=umin
  Delta : MATLAB Function  TreatAsAtomicUnit=on
  Gain : Gain  Gain=10
  Integrator : Integrator  InitialCondition=umax  LimitOutput=on  UpperSaturationLimit=umax  LowerSaturationLimit=umin
  Saturation : Saturate  UpperLimit=0.05  LowerLimit=-.2
  Saturation Dynamic : simulink/Discontinuities/Saturation Dynamic  OutMin=[]  OutMax=[]  OutDataTypeStr=Inherit: Same as second input  OutDataType=fixdt(1, 16)  OutScaling=2^-10  DoSatur=off
  Sum : Sum  Inputs=|++
  Sum1 : Sum  Inputs=-+|
  u_max : Outport
  u_saturated : Outport  Port=2
  wires:
  Gain/1 -> Saturation/1
  Sum1/1 -> Gain/1
  Sum/1 -> Sum1/2  "u+delta"
  Constant/1 -> Saturation Dynamic/3
  u_d/1 -> Saturation Dynamic/2  "ud"
  Integrator/1 -> u_max/1, Sum1/1, Saturation Dynamic/1  "umax"
  Saturation/1 -> Integrator/1
  Saturation Dynamic/1 -> Delta/1(p), Sum/1, u_saturated/1  "usat"
  Delta/1(delta) -> Sum/2

== system gensetMV/GensetAC_MVM/Genset/AVR/Low pass filter ==
  V : Inport
  Gain : Gain  Gain=1/genset.avr.T
  Integrator : Integrator  InitialCondition=genset.avr.v0
  Sum : Sum  Inputs=|+-
  Vold : Outport
  wires:
  Gain/1 -> Integrator/1
  Sum/1 -> Gain/1
  V/1 -> Sum/1
  Integrator/1 -> Sum/2, Vold/1

== system gensetMV/GensetAC_MVM/Genset/AVR/PI controller ==
  e : Inport
  Gain : Gain  Gain=genset.avr.Ki
  Gain1 : Gain  Gain=genset.avr.Kp
  Integrator : Integrator  DisableCoverage=on  InitialCondition=genset.avr.v0
  Saturation : Saturate  UpperLimit=genset.avr.max_fv  LowerLimit=genset.avr.min_fv  LinearizeAsGain=off  OutMin=genset.avr.min_fv  OutMax=genset.avr.max_fv  OutDataTypeStr=Inherit: Inherit via back propagation
  Sum : Sum  Inputs=+|+
  vf : Outport
  wires:
  Gain/1 -> Integrator/1
  Gain1/1 -> Sum/1
  Integrator/1 -> Sum/2
  e/1 -> Gain1/1, Gain/1
  Sum/1 -> Saturation/1
  Saturation/1 -> vf/1

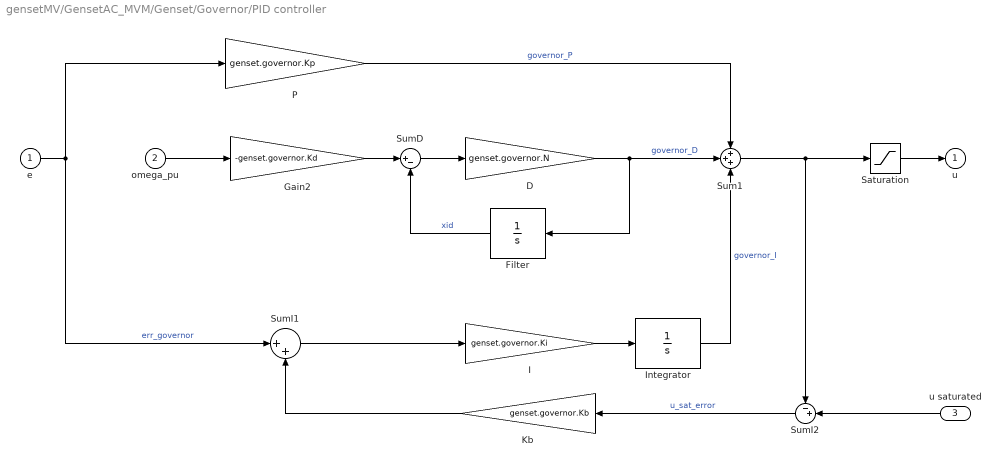
== system gensetMV/GensetAC_MVM/Genset/Governor/PID controller ==
  e : Inport  PortDimensions=1
  omega_pu : Inport  Port=2  PortDimensions=1
  u saturated : Inport  Port=3  PortDimensions=1
  D : Gain  DisableCoverage=on  Gain=genset.governor.N
  Filter : Integrator  DisableCoverage=on  InitialCondition=-genset.omega0*genset.governor.Kd
  Gain2 : Gain  Gain=-genset.governor.Kd
  I : Gain  Gain=genset.governor.Ki
  Integrator : Integrator  DisableCoverage=on  InitialCondition=genset.u0
  Kb : Gain  DisableCoverage=on  Gain=genset.governor.Kb  ParamDataTypeStr=Inherit: Inherit from 'Gain'
  P : Gain  Gain=genset.governor.Kp
  Saturation : Saturate  UpperLimit=genset.u_max  LowerLimit=genset.u_min  LinearizeAsGain=off  OutMin=genset.u_min  OutMax=genset.u_max  OutDataTypeStr=Inherit: Inherit via back propagation
  Sum1 : Sum  Inputs=+++
  SumD : Sum  DisableCoverage=on  Inputs=|+-
  SumI1 : Sum  DisableCoverage=on  Inputs=|++
  SumI2 : Sum  DisableCoverage=on  Inputs=-+|
  u : Outport  PortDimensions=1  InitialOutput=0
  wires:
  I/1 -> Integrator/1
  SumI1/1 -> I/1
  u saturated/1 -> SumI2/2
  Kb/1 -> SumI1/2
  SumI2/1 -> Kb/1  "u_sat_error"
  Sum1/1 -> SumI2/1, Saturation/1
  Gain2/1 -> SumD/1
  SumD/1 -> D/1
  Filter/1 -> SumD/2  "xid"
  Saturation/1 -> u/1
  P/1 -> Sum1/1  "governor_P"
  e/1 -> SumI1/1, P/1  "err_governor"
  omega_pu/1 -> Gain2/1
  D/1 -> Filter/1, Sum1/2  "governor_D"
  Integrator/1 -> Sum1/3  "governor_I"

== system gensetMV/GensetAC_MVM/Genset/Primover and generator/Subsystem1 ==
  d/dt : Inport
  reset : Inport  Port=2
  x0 : Inport  Port=3
  Gain : Gain  Gain=1000
  Integrator : Integrator  InitialCondition=genset.theta0
  MATLAB Function : MATLAB Function  TreatAsAtomicUnit=on
  Sum : Sum  Inputs=-|+
  Switch : Switch  Threshold=1
  Out1 : Outport
  wires:
  Switch/1 -> Integrator/1
  d/dt/1 -> Switch/1
  MATLAB Function/1(y) -> Gain/1
  Gain/1 -> Switch/3
  Sum/1 -> MATLAB Function/1(u)
  x0/1 -> Sum/2
  reset/1 -> Switch/2
  Integrator/1 -> Sum/1, Out1/1

== matlab function gensetMV/GensetDC/MATLAB Function1 ==
  data: u input
function stopper(u)
%#codegen
if ( u < -1)
    error('Bus voltage calculations have been invalid for 1 second, stopping stimulation');
end

== matlab function gensetMV/GensetAC_MVM/Genset/MATLAB Function ==
  data: Z input; connected input; p output; E input; V input; q output; Vt output
function [p,q,Vt] = power(Z,connected,E,V)
%#codegen
if (connected)
Vt = V;
V = V/sqrt(3);
s = 3*V.*conj((E-V)./Z);
p = real(s);
q = imag(s);

else
p = 0;
q = 0;
Vt =E*sqrt(3);
end

== matlab function gensetMV/GensetAC_MVM/Genset/Primover and generator/Electrical system ==
  data: umax input; p input size=1; q input; v input; genset_data input; te output; w input; pmax output size=1
function [te,pmax] = fcn(umax,p,q,v,genset_data,w)
r     = genset_data(1);
D     = genset_data(2);
p_max = genset_data(3);

te = (p+r*(p^2+q^2)/v^2)/w;
pmax = min((v/(1+r))*(-D*w^2+umax*w-r*q^2/v),p_max);

== matlab function gensetMV/Genset/MATLAB Function ==
  data: Z input; connected input; p output; E input; V input; q output; Vt output
function [p,q,Vt] = power(Z,connected,E,V)
%#codegen
if (connected)
Vt = V;
V = V/sqrt(3);
s = 3*V.*conj((E-V)./Z);
p = real(s);
q = imag(s);

else
p = 0;
q = 0;
Vt =E*sqrt(3);
end

== matlab function gensetMV/Genset/Primover and generator/Electrical system ==
  data: umax input; p input size=1; q input; v input; genset_data input; te output; w input; pmax output size=1
function [te,pmax] = fcn(umax,p,q,v,genset_data,w)
r     = genset_data(1);
D     = genset_data(2);
p_max = genset_data(3);

te = (p+r*(p^2+q^2)/v^2)/w;
pmax = min((v/(1+r))*(-D*w^2+umax*w-r*q^2/v),p_max);

== matlab function gensetMV/Genset/Primover and generator/Subsystem1/MATLAB Function ==
  data: u input; y output
function y = fcn(u)
%#codegen

y = anglemap(u);

== matlab function gensetMV/Genset/Primover and generator/turbo/MATLAB Function ==
  data: umax output; AFn parameter; ma0 parameter; AFlowcontrol parameter; u input; pin input; AF output; nr parameter
function [umax,AF] = AF(AFn,ma0,AFlowcontrol,u,pin,nr)
umax = (ma0(nr)+(1-ma0(nr))*pin)/AFlowcontrol(nr)*AFn(nr);
AF = (ma0(nr)+(1-ma0(nr))*pin)/u*AFn(nr);

== matlab function gensetMV/Genset/Primover and generator/turbo/dead-band rate limiter/Delta ==
  data: p input; delta output
function delta = fcn(p)
%#codegen
if p<.33
    delta = .33-.303*p;
elseif p<.56
    delta = .3-.217*p;
elseif p<.74
    delta = -.068+.444*p;
else
    delta = .26;
end

== matlab function gensetMV/GensetAC_MVM/Genset/Primover and generator/Subsystem1/MATLAB Function ==
  data: u input; y output
function y = fcn(u)
%#codegen

y = anglemap(u);
